simulink model "LMS_cs"  (R2023a)
settings: Solver=ode5  StartTime=0.0  StopTime=inf  FixedStep=1/200  RelTol=1e-3
PreLoadFcn:
  | mbxruntime.callbacks.PreLoadFcn(bdroot);
PostLoadFcn:
  | mbxruntime.callbacks.PostLoadFcn(bdroot);
InitFcn:
  | mbxruntime.callbacks.InitFcn(bdroot);
StartFcn:
  | mbxruntime.callbacks.StartFcn(bdroot);
StopFcn:
  | mbxruntime.callbacks.StopFcn(bdroot);
model workspace (MAT data in the model file):
  mbox_table : object (value not decoded)
  model_closed = 0
  sim_status = 0
undefined symbols (not defined in the file or in its folder): DiscIntNeverNeededParam, WheelL0, WheelL1, WheelR0, WheelR1
libraries: simulink x462, simulink_extras x117, PreScanSimulinkLibrary x33, PreScanUsefulBlocks x6, instrumentseriallib x5, simulink_need_slupdate x1
(part 4 of 68)

== system LMS_cs/BMW_X5_SUV_4 ==
  SELF_BMW_X5_SUV_4 : Inport  Tag=inport/SelfPort  OutDataTypeStr=Bus: PRESCAN_SELFSENSORDATA  PortDimensions=1  SampleTime=2/200  BusOutputAsStruct=on
  Auto_Gear : Constant  Tag=AutoGear
  Dynamics_Simple_3D : Subsystem  Tag=Simple_Vehicle_Dynamics_3D  mask(PreScan Block: Simple Dynamics 3D){Migrate=on, TimeStep=1/200, ComputationMode=Continuous_Time}
      mask prompts: Migrate "Migrate. During migration this block will be replaced by a newer one."; TimeStep "Auto assigned: Time Step [s]"; ComputationMode "Computation mode:"
      mask help:
      | The Simple Dynamics Model is selected in the GUI to simulate vehicle dynamics behavior.
      |
      | The Simple Dynamics Model is completely open to the user. The parameters of this model can be set in the Simple Dynamics dialog in the GUI.
      |
      | For more information, please click Help.
      mask init:
      | p = SimpleDyn_pars;
      settings: DeleteFcn=PreScanBlockDeleteFcn;
      mask Help: eval('openHelp(260)')
      mask Display:
      | image(imread('SimpleDyn.png'))
      | port_label('input', 1, '{\delta}_S_t_ _e_e_r [deg]','texmode','on')
      | port_label('input', 2, 'Throttle [%]')
      | port_label('input', 3, 'Brake Pres [bar]')
      | port_label('input', 4, 'V_0 [ms-1]','texmode','on')
      | port_label('input', 5, 'Auto=[0]/Manual=[1]')
      | port_label('input', 6, 'Auto_GearShift')
      | port_label('input', 7, 'Manual_GearShift')
      | port_label('input', 8, 'TyreInfo_in')
      | port_label('output', 1, 'State')
      | port_label('output', 2, 'Vx [ms-1]')
      | port_label('output', 3, 'Perf Params')
      | port_label('output', 4, 'zDispFL[m]')
      | port_label('output', 5, 'zDispFR[m]')
      | port_label('output', 6, 'zDispRL[m]')
      | port_label('output', 7, 'zDispRR[m]')
  Ground_{1..10} (10 alike) : Ground
  JointGroup_WheelDisplacement_V2R : Subsystem  Tag=mux/Wheels  mask(PreScan Velocity to Wheel Angle Block:){TimeStep=2/200, TireRadius=0.37}
      mask prompts: TimeStep "Auto Assigned: Time Step [s]"; TireRadius "Tire Radius [m]"
      settings: DeleteFcn=PreScanBlockDeleteFcn;
      mask Display: disp('Velocity\nto\nWheelAngle')
  PreScan_Contact_Sensor : Subsystem  Tag=PreScan_Contact_Sensor  LoadFcn=|  mask(PreScan Block: PreScan Contact Sensor){x0=540.252, y0=482.9517, z0=0.69, Roll0=0, Pitch0=0, Yaw0=0, wheelRadius=0.37, hcog=0.69, b=1.69, TimeStep=1/200}
      | load PrescanXYZData;
      | load PrescanRPYData;
      | load PrescanQuatData;
      | load PrescanAxisAngleData;
      | load PrescanPoseData;
      | load PrescanPoseQData;
      | load PrescanPoseAData;
      | load PrescanWheelContactData;
      mask prompts: x0 "Ini x-position VEHICLE wrt GLOBAL axis system [m]"; y0 "Ini y-position VEHICLE wrt GLOBAL axis system [m]"; z0 "Ini z-position VEHICLE wrt GLOBAL axis system [m]"; Roll0 "Ini roll-angle BODY wrt VEHICLE axis system [deg]"; Pitch0 "Ini pitch-angle BODY wrt VEHICLE axis system [deg]"; Yaw0 "Ini yaw-angle VEHICLE wrt GLOBAL axis system [deg]"; wheelRadius "Wheel Radius [m]"; hcog "Dynamics: hCoG [m]"; b "Dynamics: b [m]"; TimeStep "Time Step [s]"
      mask help:
      | This block encapsulates the base Contact sensor.
      |
      | It takes input parameters from the PreScan 3D vehicle dynamics block and outputs contact results.
      mask Help: eval('openHelp(251)')
  SELF_Demux : Subsystem  Tag=demux/SelfPort  mask(PreScan Demux Block:){}
      mask help:
      | The SELF port shows (state) information of the actor itself. The outputs are position in the experiment's axis system and the GPS coordinates, and the object's absolute velocity and compass heading.
      |
      | For more information, please click Help.
      settings: DeleteFcn=PreScanBlockDeleteFcn;
      mask Help: eval('openHelp(462)')
      mask Display:
      | port_label('output',1,'x [m]')
      | port_label('output',2,'y [m]')
      | port_label('output',3,'z [m]','texmode','on')
      | port_label('output',4,'Rotx [deg]','texmode','on')
      | port_label('output',5,'Roty [deg]','texmode','on')
      | port_label('output',6,'Rotz [deg]','texmode','on')
      | port_label('output',7,'GPS lat [deg]','texmode','on')
      | port_label('output',8,'GPS long [deg]','texmode','on')
      | port_label('output',9,'GPS alt [m]','texmode','on')
      | port_label('output',10,'Velocity [m/s]')
      | port_label('output',11,'Heading [deg]')
      | port_label('output',12,'Yaw rate [deg/s]')
  STATE_BMW_X5_SUV_4 : Subsystem  Tag=mux/StatePort  Priority=0  LoadFcn=load PrescanStateActuatorData  mask(PreScan Sink Block: State){x0=540.252, y0=482.9517, z0=0.69, Roll0=0, Pitch0=0, Yaw0=0, TimeStep=1/200}
      mask prompts: x0 "Ini x-position VEHICLE wrt GLOBAL axis system [m]"; y0 "Ini y-position VEHICLE wrt GLOBAL axis system [m]"; z0 "Ini z-position VEHICLE wrt GLOBAL axis system [m]"; Roll0 "Ini roll-angle BODY wrt VEHICLE axis system [deg]"; Pitch0 "Ini pitch-angle BODY wrt VEHICLE axis system [deg]"; Yaw0 "Ini yaw-angle VEHICLE wrt GLOBAL axis system [deg]"; TimeStep "Auto-Assigned: Upload Period [s]"
      mask help:
      | The Actor State contains a vector signal of size (9x1), containing the following signals:
      |
      | -  Position                  (x,y,z)                                     [m]
      | -  Velocity                  (vx,vy,vz)                               [m/s]
      | -  Angles                    (Roll, Pitch, Yaw)                   [rad]
      |
      | The Actor state is defined in the global axis system.
      | The state is superponed on the Initial position defined in the GUI.
      |
      | For more information, please click Help.
      settings: DeleteFcn=PreScanBlockDeleteFcn;
      mask Help: eval('openHelp(222)')
      mask Display: image(imread('State.png'))
  STATE_BMW_X5_SUV_4_rc : RateTransition  Tag=mux_rc/StatePort  OutPortSampleTimeOpt=Inherit
  Terminator_{1..13} (13 alike) : Terminator
  WheelDisplacement_Mux : Subsystem  Tag=mux/JointGroup  mask(JointGroup){}
      mask help:
      | The JointGroup allows to control several Joints in one go, as defined for this particular model.
      | For more information, look in the PreScan manual in the section "Model Preparation Tool" -> "Joint Groups"
      |
      | For more information on the Joints simulink interface, press Help.
      mask Help: eval('openHelp(254)')
  STATE_BMW_X5_SUV_4_bus : Outport  Tag=outport/StatePort  OutDataTypeStr=Bus: PRESCAN_STATEACTUATORDATA  PortDimensions=1  SampleTime=2/200
  WheelL0_BMW_X5_SUV_4 : Outport  Tag=outport/JointActuator  Port=2  OutDataTypeStr=Bus: PRESCAN_POSE_DATA  SampleTime=2/200
  WheelR0_BMW_X5_SUV_4 : Outport  Tag=outport/JointActuator  Port=3  OutDataTypeStr=Bus: PRESCAN_POSE_DATA  SampleTime=2/200
  WheelR1_BMW_X5_SUV_4 : Outport  Tag=outport/JointActuator  Port=4  OutDataTypeStr=Bus: PRESCAN_POSE_DATA  SampleTime=2/200
  WheelL1_BMW_X5_SUV_4 : Outport  Tag=outport/JointActuator  Port=5  OutDataTypeStr=Bus: PRESCAN_POSE_DATA  SampleTime=2/200
  wires:
  STATE_BMW_X5_SUV_4_rc/1 -> STATE_BMW_X5_SUV_4_bus/1
  STATE_BMW_X5_SUV_4/1(StateBus) -> STATE_BMW_X5_SUV_4_rc/1
  SELF_BMW_X5_SUV_4/1 -> SELF_Demux/1(SELF)
  WheelDisplacement_Mux/1(WheelL0_BMW_X5_SUV_4) -> WheelL0_BMW_X5_SUV_4/1
  WheelDisplacement_Mux/2(WheelR0_BMW_X5_SUV_4) -> WheelR0_BMW_X5_SUV_4/1
  WheelDisplacement_Mux/3(WheelR1_BMW_X5_SUV_4) -> WheelR1_BMW_X5_SUV_4/1
  WheelDisplacement_Mux/4(WheelL1_BMW_X5_SUV_4) -> WheelL1_BMW_X5_SUV_4/1
  JointGroup_WheelDisplacement_V2R/1(Rotation [rad]) -> WheelDisplacement_Mux/3(Rotation [rad])
  Auto_Gear/1 -> Dynamics_Simple_3D/6(Auto_GearShift)
  Dynamics_Simple_3D/8(ContactParams) -> PreScan_Contact_Sensor/1(ContactParams)
  PreScan_Contact_Sensor/1(Results) -> Dynamics_Simple_3D/8(TyreInfo_in)
  Dynamics_Simple_3D/2(Vx [m s-1]) -> JointGroup_WheelDisplacement_V2R/1(Velocity [m/s])
  Dynamics_Simple_3D/4(z_wheelFL_[m]) -> WheelDisplacement_Mux/4(zDisp FL [m])
  Dynamics_Simple_3D/5(z_wheelFR_[m]) -> WheelDisplacement_Mux/5(zDisp FR [m])
  Dynamics_Simple_3D/6(z_wheelRL_[m]) -> WheelDisplacement_Mux/6(zDisp RL [m])
  Dynamics_Simple_3D/7(z_wheelRR_[m]) -> WheelDisplacement_Mux/7(zDisp RR [m])
  Dynamics_Simple_3D/1(State) -> STATE_BMW_X5_SUV_4/1(State)
  Ground_1/1 -> Dynamics_Simple_3D/1(DeltaSteer_[deg])
  Ground_2/1 -> Dynamics_Simple_3D/2(Throttle)
  Ground_3/1 -> Dynamics_Simple_3D/3(Brake)
  Ground_4/1 -> Dynamics_Simple_3D/4(Initial_Vx_[ms-1])
  Ground_5/1 -> Dynamics_Simple_3D/5(AutoManual_OnOff)
  Ground_6/1 -> Dynamics_Simple_3D/7(Manual_GearShift)
  Dynamics_Simple_3D/3(Perf_Params) -> Terminator_1/1
  Ground_7/1 -> PreScan_Contact_Sensor/2(Steer Angle Front [deg])
  Ground_8/1 -> PreScan_Contact_Sensor/3(Steer Angle Rear [deg])
  SELF_Demux/1(x [m]) -> Terminator_2/1
  SELF_Demux/2(y [m]) -> Terminator_3/1
  SELF_Demux/3(z [m]) -> Terminator_4/1
  SELF_Demux/4(rotx [deg]) -> Terminator_5/1
  SELF_Demux/5(roty [deg]) -> Terminator_6/1
  SELF_Demux/6(rotz [deg]) -> Terminator_7/1
  SELF_Demux/7(GPS lat [deg]) -> Terminator_8/1
  SELF_Demux/8(GPS long [deg]) -> Terminator_9/1
  SELF_Demux/9(GPS alt [m]) -> Terminator_10/1
  SELF_Demux/10(velocity [m/s]) -> Terminator_11/1
  SELF_Demux/11(heading [deg]) -> Terminator_12/1
  SELF_Demux/12(yaw rate [deg/s]) -> Terminator_13/1
  Ground_9/1 -> WheelDisplacement_Mux/1(Steering Angle Front [rad])
  Ground_10/1 -> WheelDisplacement_Mux/2(Steering Angle Rear [rad])

== system LMS_cs/BMW_X5_SUV_5 ==
  SELF_BMW_X5_SUV_5 : Inport  Tag=inport/SelfPort  OutDataTypeStr=Bus: PRESCAN_SELFSENSORDATA  PortDimensions=1  SampleTime=2/200  BusOutputAsStruct=on
  Auto_Gear : Constant  Tag=AutoGear
  Dynamics_Simple_3D : Subsystem  Tag=Simple_Vehicle_Dynamics_3D  mask(PreScan Block: Simple Dynamics 3D){Migrate=on, TimeStep=1/200, ComputationMode=Continuous_Time}
      mask prompts: Migrate "Migrate. During migration this block will be replaced by a newer one."; TimeStep "Auto assigned: Time Step [s]"; ComputationMode "Computation mode:"
      mask help:
      | The Simple Dynamics Model is selected in the GUI to simulate vehicle dynamics behavior.
      |
      | The Simple Dynamics Model is completely open to the user. The parameters of this model can be set in the Simple Dynamics dialog in the GUI.
      |
      | For more information, please click Help.
      mask init:
      | p = SimpleDyn_pars;
      settings: DeleteFcn=PreScanBlockDeleteFcn;
      mask Help: eval('openHelp(260)')
      mask Display:
      | image(imread('SimpleDyn.png'))
      | port_label('input', 1, '{\delta}_S_t_ _e_e_r [deg]','texmode','on')
      | port_label('input', 2, 'Throttle [%]')
      | port_label('input', 3, 'Brake Pres [bar]')
      | port_label('input', 4, 'V_0 [ms-1]','texmode','on')
      | port_label('input', 5, 'Auto=[0]/Manual=[1]')
      | port_label('input', 6, 'Auto_GearShift')
      | port_label('input', 7, 'Manual_GearShift')
      | port_label('input', 8, 'TyreInfo_in')
      | port_label('output', 1, 'State')
      | port_label('output', 2, 'Vx [ms-1]')
      | port_label('output', 3, 'Perf Params')
      | port_label('output', 4, 'zDispFL[m]')
      | port_label('output', 5, 'zDispFR[m]')
      | port_label('output', 6, 'zDispRL[m]')
      | port_label('output', 7, 'zDispRR[m]')
  Ground_{1..10} (10 alike) : Ground
  JointGroup_WheelDisplacement_V2R : Subsystem  Tag=mux/Wheels  mask(PreScan Velocity to Wheel Angle Block:){TimeStep=2/200, TireRadius=0.37}
      mask prompts: TimeStep "Auto Assigned: Time Step [s]"; TireRadius "Tire Radius [m]"
      settings: DeleteFcn=PreScanBlockDeleteFcn;
      mask Display: disp('Velocity\nto\nWheelAngle')
  PreScan_Contact_Sensor : Subsystem  Tag=PreScan_Contact_Sensor  LoadFcn=|  mask(PreScan Block: PreScan Contact Sensor){x0=618.2031, y0=486.4632, z0=0.69, Roll0=0, Pitch0=0, Yaw0=0, wheelRadius=0.37, hcog=0.69, b=1.69, TimeStep=1/200}
      | load PrescanXYZData;
      | load PrescanRPYData;
      | load PrescanQuatData;
      | load PrescanAxisAngleData;
      | load PrescanPoseData;
      | load PrescanPoseQData;
      | load PrescanPoseAData;
      | load PrescanWheelContactData;
      mask prompts: x0 "Ini x-position VEHICLE wrt GLOBAL axis system [m]"; y0 "Ini y-position VEHICLE wrt GLOBAL axis system [m]"; z0 "Ini z-position VEHICLE wrt GLOBAL axis system [m]"; Roll0 "Ini roll-angle BODY wrt VEHICLE axis system [deg]"; Pitch0 "Ini pitch-angle BODY wrt VEHICLE axis system [deg]"; Yaw0 "Ini yaw-angle VEHICLE wrt GLOBAL axis system [deg]"; wheelRadius "Wheel Radius [m]"; hcog "Dynamics: hCoG [m]"; b "Dynamics: b [m]"; TimeStep "Time Step [s]"
      mask help:
      | This block encapsulates the base Contact sensor.
      |
      | It takes input parameters from the PreScan 3D vehicle dynamics block and outputs contact results.
      mask Help: eval('openHelp(251)')
  SELF_Demux : Subsystem  Tag=demux/SelfPort  mask(PreScan Demux Block:){}
      mask help:
      | The SELF port shows (state) information of the actor itself. The outputs are position in the experiment's axis system and the GPS coordinates, and the object's absolute velocity and compass heading.
      |
      | For more information, please click Help.
      settings: DeleteFcn=PreScanBlockDeleteFcn;
      mask Help: eval('openHelp(462)')
      mask Display:
      | port_label('output',1,'x [m]')
      | port_label('output',2,'y [m]')
      | port_label('output',3,'z [m]','texmode','on')
      | port_label('output',4,'Rotx [deg]','texmode','on')
      | port_label('output',5,'Roty [deg]','texmode','on')
      | port_label('output',6,'Rotz [deg]','texmode','on')
      | port_label('output',7,'GPS lat [deg]','texmode','on')
      | port_label('output',8,'GPS long [deg]','texmode','on')
      | port_label('output',9,'GPS alt [m]','texmode','on')
      | port_label('output',10,'Velocity [m/s]')
      | port_label('output',11,'Heading [deg]')
      | port_label('output',12,'Yaw rate [deg/s]')
  STATE_BMW_X5_SUV_5 : Subsystem  Tag=mux/StatePort  Priority=0  LoadFcn=load PrescanStateActuatorData  mask(PreScan Sink Block: State){x0=618.2031, y0=486.4632, z0=0.69, Roll0=0, Pitch0=0, Yaw0=0, TimeStep=1/200}
      mask prompts: x0 "Ini x-position VEHICLE wrt GLOBAL axis system [m]"; y0 "Ini y-position VEHICLE wrt GLOBAL axis system [m]"; z0 "Ini z-position VEHICLE wrt GLOBAL axis system [m]"; Roll0 "Ini roll-angle BODY wrt VEHICLE axis system [deg]"; Pitch0 "Ini pitch-angle BODY wrt VEHICLE axis system [deg]"; Yaw0 "Ini yaw-angle VEHICLE wrt GLOBAL axis system [deg]"; TimeStep "Auto-Assigned: Upload Period [s]"
      mask help:
      | The Actor State contains a vector signal of size (9x1), containing the following signals:
      |
      | -  Position                  (x,y,z)                                     [m]
      | -  Velocity                  (vx,vy,vz)                               [m/s]
      | -  Angles                    (Roll, Pitch, Yaw)                   [rad]
      |
      | The Actor state is defined in the global axis system.
      | The state is superponed on the Initial position defined in the GUI.
      |
      | For more information, please click Help.
      settings: DeleteFcn=PreScanBlockDeleteFcn;
      mask Help: eval('openHelp(222)')
      mask Display: image(imread('State.png'))
  STATE_BMW_X5_SUV_5_rc : RateTransition  Tag=mux_rc/StatePort  OutPortSampleTimeOpt=Inherit
  Terminator_{1..13} (13 alike) : Terminator
  WheelDisplacement_Mux : Subsystem  Tag=mux/JointGroup  mask(JointGroup){}
      mask help:
      | The JointGroup allows to control several Joints in one go, as defined for this particular model.
      | For more information, look in the PreScan manual in the section "Model Preparation Tool" -> "Joint Groups"
      |
      | For more information on the Joints simulink interface, press Help.
      mask Help: eval('openHelp(254)')
  STATE_BMW_X5_SUV_5_bus : Outport  Tag=outport/StatePort  OutDataTypeStr=Bus: PRESCAN_STATEACTUATORDATA  PortDimensions=1  SampleTime=2/200
  WheelL0_BMW_X5_SUV_5 : Outport  Tag=outport/JointActuator  Port=2  OutDataTypeStr=Bus: PRESCAN_POSE_DATA  SampleTime=2/200
  WheelR0_BMW_X5_SUV_5 : Outport  Tag=outport/JointActuator  Port=3  OutDataTypeStr=Bus: PRESCAN_POSE_DATA  SampleTime=2/200
  WheelR1_BMW_X5_SUV_5 : Outport  Tag=outport/JointActuator  Port=4  OutDataTypeStr=Bus: PRESCAN_POSE_DATA  SampleTime=2/200
  WheelL1_BMW_X5_SUV_5 : Outport  Tag=outport/JointActuator  Port=5  OutDataTypeStr=Bus: PRESCAN_POSE_DATA  SampleTime=2/200
  wires:
  STATE_BMW_X5_SUV_5_rc/1 -> STATE_BMW_X5_SUV_5_bus/1
  STATE_BMW_X5_SUV_5/1(StateBus) -> STATE_BMW_X5_SUV_5_rc/1
  SELF_BMW_X5_SUV_5/1 -> SELF_Demux/1(SELF)
  WheelDisplacement_Mux/1(WheelL0_BMW_X5_SUV_5) -> WheelL0_BMW_X5_SUV_5/1
  WheelDisplacement_Mux/2(WheelR0_BMW_X5_SUV_5) -> WheelR0_BMW_X5_SUV_5/1
  WheelDisplacement_Mux/3(WheelR1_BMW_X5_SUV_5) -> WheelR1_BMW_X5_SUV_5/1
  WheelDisplacement_Mux/4(WheelL1_BMW_X5_SUV_5) -> WheelL1_BMW_X5_SUV_5/1
  JointGroup_WheelDisplacement_V2R/1(Rotation [rad]) -> WheelDisplacement_Mux/3(Rotation [rad])
  Auto_Gear/1 -> Dynamics_Simple_3D/6(Auto_GearShift)
  Dynamics_Simple_3D/8(ContactParams) -> PreScan_Contact_Sensor/1(ContactParams)
  PreScan_Contact_Sensor/1(Results) -> Dynamics_Simple_3D/8(TyreInfo_in)
  Dynamics_Simple_3D/2(Vx [m s-1]) -> JointGroup_WheelDisplacement_V2R/1(Velocity [m/s])
  Dynamics_Simple_3D/4(z_wheelFL_[m]) -> WheelDisplacement_Mux/4(zDisp FL [m])
  Dynamics_Simple_3D/5(z_wheelFR_[m]) -> WheelDisplacement_Mux/5(zDisp FR [m])
  Dynamics_Simple_3D/6(z_wheelRL_[m]) -> WheelDisplacement_Mux/6(zDisp RL [m])
  Dynamics_Simple_3D/7(z_wheelRR_[m]) -> WheelDisplacement_Mux/7(zDisp RR [m])
  Dynamics_Simple_3D/1(State) -> STATE_BMW_X5_SUV_5/1(State)
  Ground_1/1 -> Dynamics_Simple_3D/1(DeltaSteer_[deg])
  Ground_2/1 -> Dynamics_Simple_3D/2(Throttle)
  Ground_3/1 -> Dynamics_Simple_3D/3(Brake)
  Ground_4/1 -> Dynamics_Simple_3D/4(Initial_Vx_[ms-1])
  Ground_5/1 -> Dynamics_Simple_3D/5(AutoManual_OnOff)
  Ground_6/1 -> Dynamics_Simple_3D/7(Manual_GearShift)
  Dynamics_Simple_3D/3(Perf_Params) -> Terminator_1/1
  Ground_7/1 -> PreScan_Contact_Sensor/2(Steer Angle Front [deg])
  Ground_8/1 -> PreScan_Contact_Sensor/3(Steer Angle Rear [deg])
  SELF_Demux/1(x [m]) -> Terminator_2/1
  SELF_Demux/2(y [m]) -> Terminator_3/1
  SELF_Demux/3(z [m]) -> Terminator_4/1
  SELF_Demux/4(rotx [deg]) -> Terminator_5/1
  SELF_Demux/5(roty [deg]) -> Terminator_6/1
  SELF_Demux/6(rotz [deg]) -> Terminator_7/1
  SELF_Demux/7(GPS lat [deg]) -> Terminator_8/1
  SELF_Demux/8(GPS long [deg]) -> Terminator_9/1
  SELF_Demux/9(GPS alt [m]) -> Terminator_10/1
  SELF_Demux/10(velocity [m/s]) -> Terminator_11/1
  SELF_Demux/11(heading [deg]) -> Terminator_12/1
  SELF_Demux/12(yaw rate [deg/s]) -> Terminator_13/1
  Ground_9/1 -> WheelDisplacement_Mux/1(Steering Angle Front [rad])
  Ground_10/1 -> WheelDisplacement_Mux/2(Steering Angle Rear [rad])

== system LMS_cs/BMW_X5_SUV_6 ==
  SELF_BMW_X5_SUV_6 : Inport  Tag=inport/SelfPort  OutDataTypeStr=Bus: PRESCAN_SELFSENSORDATA  PortDimensions=1  SampleTime=2/200  BusOutputAsStruct=on
  Auto_Gear : Constant  Tag=AutoGear
  Dynamics_Simple_3D : Subsystem  Tag=Simple_Vehicle_Dynamics_3D  mask(PreScan Block: Simple Dynamics 3D){Migrate=on, TimeStep=1/200, ComputationMode=Continuous_Time}
      mask prompts: Migrate "Migrate. During migration this block will be replaced by a newer one."; TimeStep "Auto assigned: Time Step [s]"; ComputationMode "Computation mode:"
      mask help:
      | The Simple Dynamics Model is selected in the GUI to simulate vehicle dynamics behavior.
      |
      | The Simple Dynamics Model is completely open to the user. The parameters of this model can be set in the Simple Dynamics dialog in the GUI.
      |
      | For more information, please click Help.
      mask init:
      | p = SimpleDyn_pars;
      settings: DeleteFcn=PreScanBlockDeleteFcn;
      mask Help: eval('openHelp(260)')
      mask Display:
      | image(imread('SimpleDyn.png'))
      | port_label('input', 1, '{\delta}_S_t_ _e_e_r [deg]','texmode','on')
      | port_label('input', 2, 'Throttle [%]')
      | port_label('input', 3, 'Brake Pres [bar]')
      | port_label('input', 4, 'V_0 [ms-1]','texmode','on')
      | port_label('input', 5, 'Auto=[0]/Manual=[1]')
      | port_label('input', 6, 'Auto_GearShift')
      | port_label('input', 7, 'Manual_GearShift')
      | port_label('input', 8, 'TyreInfo_in')
      | port_label('output', 1, 'State')
      | port_label('output', 2, 'Vx [ms-1]')
      | port_label('output', 3, 'Perf Params')
      | port_label('output', 4, 'zDispFL[m]')
      | port_label('output', 5, 'zDispFR[m]')
      | port_label('output', 6, 'zDispRL[m]')
      | port_label('output', 7, 'zDispRR[m]')
  Ground_{1..10} (10 alike) : Ground
  JointGroup_WheelDisplacement_V2R : Subsystem  Tag=mux/Wheels  mask(PreScan Velocity to Wheel Angle Block:){TimeStep=2/200, TireRadius=0.37}
      mask prompts: TimeStep "Auto Assigned: Time Step [s]"; TireRadius "Tire Radius [m]"
      settings: DeleteFcn=PreScanBlockDeleteFcn;
      mask Display: disp('Velocity\nto\nWheelAngle')
  PreScan_Contact_Sensor : Subsystem  Tag=PreScan_Contact_Sensor  LoadFcn=|  mask(PreScan Block: PreScan Contact Sensor){x0=618.2031, y0=482.8492, z0=0.69, Roll0=0, Pitch0=0, Yaw0=0, wheelRadius=0.37, hcog=0.69, b=1.69, TimeStep=1/200}
      | load PrescanXYZData;
      | load PrescanRPYData;
      | load PrescanQuatData;
      | load PrescanAxisAngleData;
      | load PrescanPoseData;
      | load PrescanPoseQData;
      | load PrescanPoseAData;
      | load PrescanWheelContactData;
      mask prompts: x0 "Ini x-position VEHICLE wrt GLOBAL axis system [m]"; y0 "Ini y-position VEHICLE wrt GLOBAL axis system [m]"; z0 "Ini z-position VEHICLE wrt GLOBAL axis system [m]"; Roll0 "Ini roll-angle BODY wrt VEHICLE axis system [deg]"; Pitch0 "Ini pitch-angle BODY wrt VEHICLE axis system [deg]"; Yaw0 "Ini yaw-angle VEHICLE wrt GLOBAL axis system [deg]"; wheelRadius "Wheel Radius [m]"; hcog "Dynamics: hCoG [m]"; b "Dynamics: b [m]"; TimeStep "Time Step [s]"
      mask help:
      | This block encapsulates the base Contact sensor.
      |
      | It takes input parameters from the PreScan 3D vehicle dynamics block and outputs contact results.
      mask Help: eval('openHelp(251)')
  SELF_Demux : Subsystem  Tag=demux/SelfPort  mask(PreScan Demux Block:){}
      mask help:
      | The SELF port shows (state) information of the actor itself. The outputs are position in the experiment's axis system and the GPS coordinates, and the object's absolute velocity and compass heading.
      |
      | For more information, please click Help.
      settings: DeleteFcn=PreScanBlockDeleteFcn;
      mask Help: eval('openHelp(462)')
      mask Display:
      | port_label('output',1,'x [m]')
      | port_label('output',2,'y [m]')
      | port_label('output',3,'z [m]','texmode','on')
      | port_label('output',4,'Rotx [deg]','texmode','on')
      | port_label('output',5,'Roty [deg]','texmode','on')
      | port_label('output',6,'Rotz [deg]','texmode','on')
      | port_label('output',7,'GPS lat [deg]','texmode','on')
      | port_label('output',8,'GPS long [deg]','texmode','on')
      | port_label('output',9,'GPS alt [m]','texmode','on')
      | port_label('output',10,'Velocity [m/s]')
      | port_label('output',11,'Heading [deg]')
      | port_label('output',12,'Yaw rate [deg/s]')
  STATE_BMW_X5_SUV_6 : Subsystem  Tag=mux/StatePort  Priority=0  LoadFcn=load PrescanStateActuatorData  mask(PreScan Sink Block: State){x0=618.2031, y0=482.8492, z0=0.69, Roll0=0, Pitch0=0, Yaw0=0, TimeStep=1/200}
      mask prompts: x0 "Ini x-position VEHICLE wrt GLOBAL axis system [m]"; y0 "Ini y-position VEHICLE wrt GLOBAL axis system [m]"; z0 "Ini z-position VEHICLE wrt GLOBAL axis system [m]"; Roll0 "Ini roll-angle BODY wrt VEHICLE axis system [deg]"; Pitch0 "Ini pitch-angle BODY wrt VEHICLE axis system [deg]"; Yaw0 "Ini yaw-angle VEHICLE wrt GLOBAL axis system [deg]"; TimeStep "Auto-Assigned: Upload Period [s]"
      mask help:
      | The Actor State contains a vector signal of size (9x1), containing the following signals:
      |
      | -  Position                  (x,y,z)                                     [m]
      | -  Velocity                  (vx,vy,vz)                               [m/s]
      | -  Angles                    (Roll, Pitch, Yaw)                   [rad]
      |
      | The Actor state is defined in the global axis system.
      | The state is superponed on the Initial position defined in the GUI.
      |
      | For more information, please click Help.
      settings: DeleteFcn=PreScanBlockDeleteFcn;
      mask Help: eval('openHelp(222)')
      mask Display: image(imread('State.png'))
  STATE_BMW_X5_SUV_6_rc : RateTransition  Tag=mux_rc/StatePort  OutPortSampleTimeOpt=Inherit
  Terminator_{1..13} (13 alike) : Terminator
  WheelDisplacement_Mux : Subsystem  Tag=mux/JointGroup  mask(JointGroup){}
      mask help:
      | The JointGroup allows to control several Joints in one go, as defined for this particular model.
      | For more information, look in the PreScan manual in the section "Model Preparation Tool" -> "Joint Groups"
      |
      | For more information on the Joints simulink interface, press Help.
      mask Help: eval('openHelp(254)')
  STATE_BMW_X5_SUV_6_bus : Outport  Tag=outport/StatePort  OutDataTypeStr=Bus: PRESCAN_STATEACTUATORDATA  PortDimensions=1  SampleTime=2/200
  WheelL0_BMW_X5_SUV_6 : Outport  Tag=outport/JointActuator  Port=2  OutDataTypeStr=Bus: PRESCAN_POSE_DATA  SampleTime=2/200
  WheelR0_BMW_X5_SUV_6 : Outport  Tag=outport/JointActuator  Port=3  OutDataTypeStr=Bus: PRESCAN_POSE_DATA  SampleTime=2/200
  WheelR1_BMW_X5_SUV_6 : Outport  Tag=outport/JointActuator  Port=4  OutDataTypeStr=Bus: PRESCAN_POSE_DATA  SampleTime=2/200
  WheelL1_BMW_X5_SUV_6 : Outport  Tag=outport/JointActuator  Port=5  OutDataTypeStr=Bus: PRESCAN_POSE_DATA  SampleTime=2/200
  wires:
  STATE_BMW_X5_SUV_6_rc/1 -> STATE_BMW_X5_SUV_6_bus/1
  STATE_BMW_X5_SUV_6/1(StateBus) -> STATE_BMW_X5_SUV_6_rc/1
  SELF_BMW_X5_SUV_6/1 -> SELF_Demux/1(SELF)
  WheelDisplacement_Mux/1(WheelL0_BMW_X5_SUV_6) -> WheelL0_BMW_X5_SUV_6/1
  WheelDisplacement_Mux/2(WheelR0_BMW_X5_SUV_6) -> WheelR0_BMW_X5_SUV_6/1
  WheelDisplacement_Mux/3(WheelR1_BMW_X5_SUV_6) -> WheelR1_BMW_X5_SUV_6/1
  WheelDisplacement_Mux/4(WheelL1_BMW_X5_SUV_6) -> WheelL1_BMW_X5_SUV_6/1
  JointGroup_WheelDisplacement_V2R/1(Rotation [rad]) -> WheelDisplacement_Mux/3(Rotation [rad])
  Auto_Gear/1 -> Dynamics_Simple_3D/6(Auto_GearShift)
  Dynamics_Simple_3D/8(ContactParams) -> PreScan_Contact_Sensor/1(ContactParams)
  PreScan_Contact_Sensor/1(Results) -> Dynamics_Simple_3D/8(TyreInfo_in)
  Dynamics_Simple_3D/2(Vx [m s-1]) -> JointGroup_WheelDisplacement_V2R/1(Velocity [m/s])
  Dynamics_Simple_3D/4(z_wheelFL_[m]) -> WheelDisplacement_Mux/4(zDisp FL [m])
  Dynamics_Simple_3D/5(z_wheelFR_[m]) -> WheelDisplacement_Mux/5(zDisp FR [m])
  Dynamics_Simple_3D/6(z_wheelRL_[m]) -> WheelDisplacement_Mux/6(zDisp RL [m])
  Dynamics_Simple_3D/7(z_wheelRR_[m]) -> WheelDisplacement_Mux/7(zDisp RR [m])
  Dynamics_Simple_3D/1(State) -> STATE_BMW_X5_SUV_6/1(State)
  Ground_1/1 -> Dynamics_Simple_3D/1(DeltaSteer_[deg])
  Ground_2/1 -> Dynamics_Simple_3D/2(Throttle)
  Ground_3/1 -> Dynamics_Simple_3D/3(Brake)
  Ground_4/1 -> Dynamics_Simple_3D/4(Initial_Vx_[ms-1])
  Ground_5/1 -> Dynamics_Simple_3D/5(AutoManual_OnOff)
  Ground_6/1 -> Dynamics_Simple_3D/7(Manual_GearShift)
  Dynamics_Simple_3D/3(Perf_Params) -> Terminator_1/1
  Ground_7/1 -> PreScan_Contact_Sensor/2(Steer Angle Front [deg])
  Ground_8/1 -> PreScan_Contact_Sensor/3(Steer Angle Rear [deg])
  SELF_Demux/1(x [m]) -> Terminator_2/1
  SELF_Demux/2(y [m]) -> Terminator_3/1
  SELF_Demux/3(z [m]) -> Terminator_4/1
  SELF_Demux/4(rotx [deg]) -> Terminator_5/1
  SELF_Demux/5(roty [deg]) -> Terminator_6/1
  SELF_Demux/6(rotz [deg]) -> Terminator_7/1
  SELF_Demux/7(GPS lat [deg]) -> Terminator_8/1
  SELF_Demux/8(GPS long [deg]) -> Terminator_9/1
  SELF_Demux/9(GPS alt [m]) -> Terminator_10/1
  SELF_Demux/10(velocity [m/s]) -> Terminator_11/1
  SELF_Demux/11(heading [deg]) -> Terminator_12/1
  SELF_Demux/12(yaw rate [deg/s]) -> Terminator_13/1
  Ground_9/1 -> WheelDisplacement_Mux/1(Steering Angle Front [rad])
  Ground_10/1 -> WheelDisplacement_Mux/2(Steering Angle Rear [rad])

== system LMS_cs/BMW_X5_SUV_7 ==
  SELF_BMW_X5_SUV_7 : Inport  Tag=inport/SelfPort  OutDataTypeStr=Bus: PRESCAN_SELFSENSORDATA  PortDimensions=1  SampleTime=2/200  BusOutputAsStruct=on
  Auto_Gear : Constant  Tag=AutoGear
  Dynamics_Simple_3D : Subsystem  Tag=Simple_Vehicle_Dynamics_3D  mask(PreScan Block: Simple Dynamics 3D){Migrate=on, TimeStep=1/200, ComputationMode=Continuous_Time}
      mask prompts: Migrate "Migrate. During migration this block will be replaced by a newer one."; TimeStep "Auto assigned: Time Step [s]"; ComputationMode "Computation mode:"
      mask help:
      | The Simple Dynamics Model is selected in the GUI to simulate vehicle dynamics behavior.
      |
      | The Simple Dynamics Model is completely open to the user. The parameters of this model can be set in the Simple Dynamics dialog in the GUI.
      |
      | For more information, please click Help.
      mask init:
      | p = SimpleDyn_pars;
      settings: DeleteFcn=PreScanBlockDeleteFcn;
      mask Help: eval('openHelp(260)')
      mask Display:
      | image(imread('SimpleDyn.png'))
      | port_label('input', 1, '{\delta}_S_t_ _e_e_r [deg]','texmode','on')
      | port_label('input', 2, 'Throttle [%]')
      | port_label('input', 3, 'Brake Pres [bar]')
      | port_label('input', 4, 'V_0 [ms-1]','texmode','on')
      | port_label('input', 5, 'Auto=[0]/Manual=[1]')
      | port_label('input', 6, 'Auto_GearShift')
      | port_label('input', 7, 'Manual_GearShift')
      | port_label('input', 8, 'TyreInfo_in')
      | port_label('output', 1, 'State')
      | port_label('output', 2, 'Vx [ms-1]')
      | port_label('output', 3, 'Perf Params')
      | port_label('output', 4, 'zDispFL[m]')
      | port_label('output', 5, 'zDispFR[m]')
      | port_label('output', 6, 'zDispRL[m]')
      | port_label('output', 7, 'zDispRR[m]')
  Ground_{1..10} (10 alike) : Ground
  JointGroup_WheelDisplacement_V2R : Subsystem  Tag=mux/Wheels  mask(PreScan Velocity to Wheel Angle Block:){TimeStep=2/200, TireRadius=0.37}
      mask prompts: TimeStep "Auto Assigned: Time Step [s]"; TireRadius "Tire Radius [m]"
      settings: DeleteFcn=PreScanBlockDeleteFcn;
      mask Display: disp('Velocity\nto\nWheelAngle')
  PreScan_Contact_Sensor : Subsystem  Tag=PreScan_Contact_Sensor  LoadFcn=|  mask(PreScan Block: PreScan Contact Sensor){x0=699.4634, y0=489.8891, z0=0.69, Roll0=0, Pitch0=0, Yaw0=0, wheelRadius=0.37, hcog=0.69, b=1.69, TimeStep=1/200}
      | load PrescanXYZData;
      | load PrescanRPYData;
      | load PrescanQuatData;
      | load PrescanAxisAngleData;
      | load PrescanPoseData;
      | load PrescanPoseQData;
      | load PrescanPoseAData;
      | load PrescanWheelContactData;
      mask prompts: x0 "Ini x-position VEHICLE wrt GLOBAL axis system [m]"; y0 "Ini y-position VEHICLE wrt GLOBAL axis system [m]"; z0 "Ini z-position VEHICLE wrt GLOBAL axis system [m]"; Roll0 "Ini roll-angle BODY wrt VEHICLE axis system [deg]"; Pitch0 "Ini pitch-angle BODY wrt VEHICLE axis system [deg]"; Yaw0 "Ini yaw-angle VEHICLE wrt GLOBAL axis system [deg]"; wheelRadius "Wheel Radius [m]"; hcog "Dynamics: hCoG [m]"; b "Dynamics: b [m]"; TimeStep "Time Step [s]"
      mask help:
      | This block encapsulates the base Contact sensor.
      |
      | It takes input parameters from the PreScan 3D vehicle dynamics block and outputs contact results.
      mask Help: eval('openHelp(251)')
  SELF_Demux : Subsystem  Tag=demux/SelfPort  mask(PreScan Demux Block:){}
      mask help:
      | The SELF port shows (state) information of the actor itself. The outputs are position in the experiment's axis system and the GPS coordinates, and the object's absolute velocity and compass heading.
      |
      | For more information, please click Help.
      settings: DeleteFcn=PreScanBlockDeleteFcn;
      mask Help: eval('openHelp(462)')
      mask Display:
      | port_label('output',1,'x [m]')
      | port_label('output',2,'y [m]')
      | port_label('output',3,'z [m]','texmode','on')
      | port_label('output',4,'Rotx [deg]','texmode','on')
      | port_label('output',5,'Roty [deg]','texmode','on')
      | port_label('output',6,'Rotz [deg]','texmode','on')
      | port_label('output',7,'GPS lat [deg]','texmode','on')
      | port_label('output',8,'GPS long [deg]','texmode','on')
      | port_label('output',9,'GPS alt [m]','texmode','on')
      | port_label('output',10,'Velocity [m/s]')
      | port_label('output',11,'Heading [deg]')
      | port_label('output',12,'Yaw rate [deg/s]')
  STATE_BMW_X5_SUV_7 : Subsystem  Tag=mux/StatePort  Priority=0  LoadFcn=load PrescanStateActuatorData  mask(PreScan Sink Block: State){x0=699.4634, y0=489.8891, z0=0.69, Roll0=0, Pitch0=0, Yaw0=0, TimeStep=1/200}
      mask prompts: x0 "Ini x-position VEHICLE wrt GLOBAL axis system [m]"; y0 "Ini y-position VEHICLE wrt GLOBAL axis system [m]"; z0 "Ini z-position VEHICLE wrt GLOBAL axis system [m]"; Roll0 "Ini roll-angle BODY wrt VEHICLE axis system [deg]"; Pitch0 "Ini pitch-angle BODY wrt VEHICLE axis system [deg]"; Yaw0 "Ini yaw-angle VEHICLE wrt GLOBAL axis system [deg]"; TimeStep "Auto-Assigned: Upload Period [s]"
      mask help:
      | The Actor State contains a vector signal of size (9x1), containing the following signals:
      |
      | -  Position                  (x,y,z)                                     [m]
      | -  Velocity                  (vx,vy,vz)                               [m/s]
      | -  Angles                    (Roll, Pitch, Yaw)                   [rad]
      |
      | The Actor state is defined in the global axis system.
      | The state is superponed on the Initial position defined in the GUI.
      |
      | For more information, please click Help.
      settings: DeleteFcn=PreScanBlockDeleteFcn;
      mask Help: eval('openHelp(222)')
      mask Display: image(imread('State.png'))
  STATE_BMW_X5_SUV_7_rc : RateTransition  Tag=mux_rc/StatePort  OutPortSampleTimeOpt=Inherit
  Terminator_{1..13} (13 alike) : Terminator
  WheelDisplacement_Mux : Subsystem  Tag=mux/JointGroup  mask(JointGroup){}
      mask help:
      | The JointGroup allows to control several Joints in one go, as defined for this particular model.
      | For more information, look in the PreScan manual in the section "Model Preparation Tool" -> "Joint Groups"
      |
      | For more information on the Joints simulink interface, press Help.
      mask Help: eval('openHelp(254)')
  STATE_BMW_X5_SUV_7_bus : Outport  Tag=outport/StatePort  OutDataTypeStr=Bus: PRESCAN_STATEACTUATORDATA  PortDimensions=1  SampleTime=2/200
  WheelL0_BMW_X5_SUV_7 : Outport  Tag=outport/JointActuator  Port=2  OutDataTypeStr=Bus: PRESCAN_POSE_DATA  SampleTime=2/200
  WheelR0_BMW_X5_SUV_7 : Outport  Tag=outport/JointActuator  Port=3  OutDataTypeStr=Bus: PRESCAN_POSE_DATA  SampleTime=2/200
  WheelR1_BMW_X5_SUV_7 : Outport  Tag=outport/JointActuator  Port=4  OutDataTypeStr=Bus: PRESCAN_POSE_DATA  SampleTime=2/200
  WheelL1_BMW_X5_SUV_7 : Outport  Tag=outport/JointActuator  Port=5  OutDataTypeStr=Bus: PRESCAN_POSE_DATA  SampleTime=2/200
  wires:
  STATE_BMW_X5_SUV_7_rc/1 -> STATE_BMW_X5_SUV_7_bus/1
  STATE_BMW_X5_SUV_7/1(StateBus) -> STATE_BMW_X5_SUV_7_rc/1
  SELF_BMW_X5_SUV_7/1 -> SELF_Demux/1(SELF)
  WheelDisplacement_Mux/1(WheelL0_BMW_X5_SUV_7) -> WheelL0_BMW_X5_SUV_7/1
  WheelDisplacement_Mux/2(WheelR0_BMW_X5_SUV_7) -> WheelR0_BMW_X5_SUV_7/1
  WheelDisplacement_Mux/3(WheelR1_BMW_X5_SUV_7) -> WheelR1_BMW_X5_SUV_7/1
  WheelDisplacement_Mux/4(WheelL1_BMW_X5_SUV_7) -> WheelL1_BMW_X5_SUV_7/1
  JointGroup_WheelDisplacement_V2R/1(Rotation [rad]) -> WheelDisplacement_Mux/3(Rotation [rad])
  Auto_Gear/1 -> Dynamics_Simple_3D/6(Auto_GearShift)
  Dynamics_Simple_3D/8(ContactParams) -> PreScan_Contact_Sensor/1(ContactParams)
  PreScan_Contact_Sensor/1(Results) -> Dynamics_Simple_3D/8(TyreInfo_in)
  Dynamics_Simple_3D/2(Vx [m s-1]) -> JointGroup_WheelDisplacement_V2R/1(Velocity [m/s])
  Dynamics_Simple_3D/4(z_wheelFL_[m]) -> WheelDisplacement_Mux/4(zDisp FL [m])
  Dynamics_Simple_3D/5(z_wheelFR_[m]) -> WheelDisplacement_Mux/5(zDisp FR [m])
  Dynamics_Simple_3D/6(z_wheelRL_[m]) -> WheelDisplacement_Mux/6(zDisp RL [m])
  Dynamics_Simple_3D/7(z_wheelRR_[m]) -> WheelDisplacement_Mux/7(zDisp RR [m])
  Dynamics_Simple_3D/1(State) -> STATE_BMW_X5_SUV_7/1(State)
  Ground_1/1 -> Dynamics_Simple_3D/1(DeltaSteer_[deg])
  Ground_2/1 -> Dynamics_Simple_3D/2(Throttle)
  Ground_3/1 -> Dynamics_Simple_3D/3(Brake)
  Ground_4/1 -> Dynamics_Simple_3D/4(Initial_Vx_[ms-1])
  Ground_5/1 -> Dynamics_Simple_3D/5(AutoManual_OnOff)
  Ground_6/1 -> Dynamics_Simple_3D/7(Manual_GearShift)
  Dynamics_Simple_3D/3(Perf_Params) -> Terminator_1/1
  Ground_7/1 -> PreScan_Contact_Sensor/2(Steer Angle Front [deg])
  Ground_8/1 -> PreScan_Contact_Sensor/3(Steer Angle Rear [deg])
  SELF_Demux/1(x [m]) -> Terminator_2/1
  SELF_Demux/2(y [m]) -> Terminator_3/1
  SELF_Demux/3(z [m]) -> Terminator_4/1
  SELF_Demux/4(rotx [deg]) -> Terminator_5/1
  SELF_Demux/5(roty [deg]) -> Terminator_6/1
  SELF_Demux/6(rotz [deg]) -> Terminator_7/1
  SELF_Demux/7(GPS lat [deg]) -> Terminator_8/1
  SELF_Demux/8(GPS long [deg]) -> Terminator_9/1
  SELF_Demux/9(GPS alt [m]) -> Terminator_10/1
  SELF_Demux/10(velocity [m/s]) -> Terminator_11/1
  SELF_Demux/11(heading [deg]) -> Terminator_12/1
  SELF_Demux/12(yaw rate [deg/s]) -> Terminator_13/1
  Ground_9/1 -> WheelDisplacement_Mux/1(Steering Angle Front [rad])
  Ground_10/1 -> WheelDisplacement_Mux/2(Steering Angle Rear [rad])

== system LMS_cs/BMW_X5_SUV_8 ==
  SELF_BMW_X5_SUV_8 : Inport  Tag=inport/SelfPort  OutDataTypeStr=Bus: PRESCAN_SELFSENSORDATA  PortDimensions=1  SampleTime=2/200  BusOutputAsStruct=on
  Auto_Gear : Constant  Tag=AutoGear
  Dynamics_Simple_3D : Subsystem  Tag=Simple_Vehicle_Dynamics_3D  mask(PreScan Block: Simple Dynamics 3D){Migrate=on, TimeStep=1/200, ComputationMode=Continuous_Time}
      mask prompts: Migrate "Migrate. During migration this block will be replaced by a newer one."; TimeStep "Auto assigned: Time Step [s]"; ComputationMode "Computation mode:"
      mask help:
      | The Simple Dynamics Model is selected in the GUI to simulate vehicle dynamics behavior.
      |
      | The Simple Dynamics Model is completely open to the user. The parameters of this model can be set in the Simple Dynamics dialog in the GUI.
      |
      | For more information, please click Help.
      mask init:
      | p = SimpleDyn_pars;
      settings: DeleteFcn=PreScanBlockDeleteFcn;
      mask Help: eval('openHelp(260)')
      mask Display:
      | image(imread('SimpleDyn.png'))
      | port_label('input', 1, '{\delta}_S_t_ _e_e_r [deg]','texmode','on')
      | port_label('input', 2, 'Throttle [%]')
      | port_label('input', 3, 'Brake Pres [bar]')
      | port_label('input', 4, 'V_0 [ms-1]','texmode','on')
      | port_label('input', 5, 'Auto=[0]/Manual=[1]')
      | port_label('input', 6, 'Auto_GearShift')
      | port_label('input', 7, 'Manual_GearShift')
      | port_label('input', 8, 'TyreInfo_in')
      | port_label('output', 1, 'State')
      | port_label('output', 2, 'Vx [ms-1]')
      | port_label('output', 3, 'Perf Params')
      | port_label('output', 4, 'zDispFL[m]')
      | port_label('output', 5, 'zDispFR[m]')
      | port_label('output', 6, 'zDispRL[m]')
      | port_label('output', 7, 'zDispRR[m]')
  Ground_{1..10} (10 alike) : Ground
  JointGroup_WheelDisplacement_V2R : Subsystem  Tag=mux/Wheels  mask(PreScan Velocity to Wheel Angle Block:){TimeStep=2/200, TireRadius=0.37}
      mask prompts: TimeStep "Auto Assigned: Time Step [s]"; TireRadius "Tire Radius [m]"
      settings: DeleteFcn=PreScanBlockDeleteFcn;
      mask Display: disp('Velocity\nto\nWheelAngle')
  PreScan_Contact_Sensor : Subsystem  Tag=PreScan_Contact_Sensor  LoadFcn=|  mask(PreScan Block: PreScan Contact Sensor){x0=746.4608, y0=486.4069, z0=0.69, Roll0=0, Pitch0=0, Yaw0=0, wheelRadius=0.37, hcog=0.69, b=1.69, TimeStep=1/200}
      | load PrescanXYZData;
      | load PrescanRPYData;
      | load PrescanQuatData;
      | load PrescanAxisAngleData;
      | load PrescanPoseData;
      | load PrescanPoseQData;
      | load PrescanPoseAData;
      | load PrescanWheelContactData;
      mask prompts: x0 "Ini x-position VEHICLE wrt GLOBAL axis system [m]"; y0 "Ini y-position VEHICLE wrt GLOBAL axis system [m]"; z0 "Ini z-position VEHICLE wrt GLOBAL axis system [m]"; Roll0 "Ini roll-angle BODY wrt VEHICLE axis system [deg]"; Pitch0 "Ini pitch-angle BODY wrt VEHICLE axis system [deg]"; Yaw0 "Ini yaw-angle VEHICLE wrt GLOBAL axis system [deg]"; wheelRadius "Wheel Radius [m]"; hcog "Dynamics: hCoG [m]"; b "Dynamics: b [m]"; TimeStep "Time Step [s]"
      mask help:
      | This block encapsulates the base Contact sensor.
      |
      | It takes input parameters from the PreScan 3D vehicle dynamics block and outputs contact results.
      mask Help: eval('openHelp(251)')
  SELF_Demux : Subsystem  Tag=demux/SelfPort  mask(PreScan Demux Block:){}
      mask help:
      | The SELF port shows (state) information of the actor itself. The outputs are position in the experiment's axis system and the GPS coordinates, and the object's absolute velocity and compass heading.
      |
      | For more information, please click Help.
      settings: DeleteFcn=PreScanBlockDeleteFcn;
      mask Help: eval('openHelp(462)')
      mask Display:
      | port_label('output',1,'x [m]')
      | port_label('output',2,'y [m]')
      | port_label('output',3,'z [m]','texmode','on')
      | port_label('output',4,'Rotx [deg]','texmode','on')
      | port_label('output',5,'Roty [deg]','texmode','on')
      | port_label('output',6,'Rotz [deg]','texmode','on')
      | port_label('output',7,'GPS lat [deg]','texmode','on')
      | port_label('output',8,'GPS long [deg]','texmode','on')
      | port_label('output',9,'GPS alt [m]','texmode','on')
      | port_label('output',10,'Velocity [m/s]')
      | port_label('output',11,'Heading [deg]')
      | port_label('output',12,'Yaw rate [deg/s]')
  STATE_BMW_X5_SUV_8 : Subsystem  Tag=mux/StatePort  Priority=0  LoadFcn=load PrescanStateActuatorData  mask(PreScan Sink Block: State){x0=746.4608, y0=486.4069, z0=0.69, Roll0=0, Pitch0=0, Yaw0=0, TimeStep=1/200}
      mask prompts: x0 "Ini x-position VEHICLE wrt GLOBAL axis system [m]"; y0 "Ini y-position VEHICLE wrt GLOBAL axis system [m]"; z0 "Ini z-position VEHICLE wrt GLOBAL axis system [m]"; Roll0 "Ini roll-angle BODY wrt VEHICLE axis system [deg]"; Pitch0 "Ini pitch-angle BODY wrt VEHICLE axis system [deg]"; Yaw0 "Ini yaw-angle VEHICLE wrt GLOBAL axis system [deg]"; TimeStep "Auto-Assigned: Upload Period [s]"
      mask help:
      | The Actor State contains a vector signal of size (9x1), containing the following signals:
      |
      | -  Position                  (x,y,z)                                     [m]
      | -  Velocity                  (vx,vy,vz)                               [m/s]
      | -  Angles                    (Roll, Pitch, Yaw)                   [rad]
      |
      | The Actor state is defined in the global axis system.
      | The state is superponed on the Initial position defined in the GUI.
      |
      | For more information, please click Help.
      settings: DeleteFcn=PreScanBlockDeleteFcn;
      mask Help: eval('openHelp(222)')
      mask Display: image(imread('State.png'))
  STATE_BMW_X5_SUV_8_rc : RateTransition  Tag=mux_rc/StatePort  OutPortSampleTimeOpt=Inherit
  Terminator_{1..13} (13 alike) : Terminator
  WheelDisplacement_Mux : Subsystem  Tag=mux/JointGroup  mask(JointGroup){}
      mask help:
      | The JointGroup allows to control several Joints in one go, as defined for this particular model.
      | For more information, look in the PreScan manual in the section "Model Preparation Tool" -> "Joint Groups"
      |
      | For more information on the Joints simulink interface, press Help.
      mask Help: eval('openHelp(254)')
  STATE_BMW_X5_SUV_8_bus : Outport  Tag=outport/StatePort  OutDataTypeStr=Bus: PRESCAN_STATEACTUATORDATA  PortDimensions=1  SampleTime=2/200
  WheelL0_BMW_X5_SUV_8 : Outport  Tag=outport/JointActuator  Port=2  OutDataTypeStr=Bus: PRESCAN_POSE_DATA  SampleTime=2/200
  WheelR0_BMW_X5_SUV_8 : Outport  Tag=outport/JointActuator  Port=3  OutDataTypeStr=Bus: PRESCAN_POSE_DATA  SampleTime=2/200
  WheelR1_BMW_X5_SUV_8 : Outport  Tag=outport/JointActuator  Port=4  OutDataTypeStr=Bus: PRESCAN_POSE_DATA  SampleTime=2/200
  WheelL1_BMW_X5_SUV_8 : Outport  Tag=outport/JointActuator  Port=5  OutDataTypeStr=Bus: PRESCAN_POSE_DATA  SampleTime=2/200
  wires:
  STATE_BMW_X5_SUV_8_rc/1 -> STATE_BMW_X5_SUV_8_bus/1
  STATE_BMW_X5_SUV_8/1(StateBus) -> STATE_BMW_X5_SUV_8_rc/1
  SELF_BMW_X5_SUV_8/1 -> SELF_Demux/1(SELF)
  WheelDisplacement_Mux/1(WheelL0_BMW_X5_SUV_8) -> WheelL0_BMW_X5_SUV_8/1
  WheelDisplacement_Mux/2(WheelR0_BMW_X5_SUV_8) -> WheelR0_BMW_X5_SUV_8/1
  WheelDisplacement_Mux/3(WheelR1_BMW_X5_SUV_8) -> WheelR1_BMW_X5_SUV_8/1
  WheelDisplacement_Mux/4(WheelL1_BMW_X5_SUV_8) -> WheelL1_BMW_X5_SUV_8/1
  JointGroup_WheelDisplacement_V2R/1(Rotation [rad]) -> WheelDisplacement_Mux/3(Rotation [rad])
  Auto_Gear/1 -> Dynamics_Simple_3D/6(Auto_GearShift)
  Dynamics_Simple_3D/8(ContactParams) -> PreScan_Contact_Sensor/1(ContactParams)
  PreScan_Contact_Sensor/1(Results) -> Dynamics_Simple_3D/8(TyreInfo_in)
  Dynamics_Simple_3D/2(Vx [m s-1]) -> JointGroup_WheelDisplacement_V2R/1(Velocity [m/s])
  Dynamics_Simple_3D/4(z_wheelFL_[m]) -> WheelDisplacement_Mux/4(zDisp FL [m])
  Dynamics_Simple_3D/5(z_wheelFR_[m]) -> WheelDisplacement_Mux/5(zDisp FR [m])
  Dynamics_Simple_3D/6(z_wheelRL_[m]) -> WheelDisplacement_Mux/6(zDisp RL [m])
  Dynamics_Simple_3D/7(z_wheelRR_[m]) -> WheelDisplacement_Mux/7(zDisp RR [m])
  Dynamics_Simple_3D/1(State) -> STATE_BMW_X5_SUV_8/1(State)
  Ground_1/1 -> Dynamics_Simple_3D/1(DeltaSteer_[deg])
  Ground_2/1 -> Dynamics_Simple_3D/2(Throttle)
  Ground_3/1 -> Dynamics_Simple_3D/3(Brake)
  Ground_4/1 -> Dynamics_Simple_3D/4(Initial_Vx_[ms-1])
  Ground_5/1 -> Dynamics_Simple_3D/5(AutoManual_OnOff)
  Ground_6/1 -> Dynamics_Simple_3D/7(Manual_GearShift)
  Dynamics_Simple_3D/3(Perf_Params) -> Terminator_1/1
  Ground_7/1 -> PreScan_Contact_Sensor/2(Steer Angle Front [deg])
  Ground_8/1 -> PreScan_Contact_Sensor/3(Steer Angle Rear [deg])
  SELF_Demux/1(x [m]) -> Terminator_2/1
  SELF_Demux/2(y [m]) -> Terminator_3/1
  SELF_Demux/3(z [m]) -> Terminator_4/1
  SELF_Demux/4(rotx [deg]) -> Terminator_5/1
  SELF_Demux/5(roty [deg]) -> Terminator_6/1
  SELF_Demux/6(rotz [deg]) -> Terminator_7/1
  SELF_Demux/7(GPS lat [deg]) -> Terminator_8/1
  SELF_Demux/8(GPS long [deg]) -> Terminator_9/1
  SELF_Demux/9(GPS alt [m]) -> Terminator_10/1
  SELF_Demux/10(velocity [m/s]) -> Terminator_11/1
  SELF_Demux/11(heading [deg]) -> Terminator_12/1
  SELF_Demux/12(yaw rate [deg/s]) -> Terminator_13/1
  Ground_9/1 -> WheelDisplacement_Mux/1(Steering Angle Front [rad])
  Ground_10/1 -> WheelDisplacement_Mux/2(Steering Angle Rear [rad])
